simulink model "Orig_DSR_mod"  (R2021a)
settings: Solver=VariableStepAuto  StartTime=0.0  StopTime=10  RelTol=1e-3
values from neighbouring files (symbols this model uses):
  a = 0.5    [plot_3.m]
  alpha = 1.192    [plot_3.m]
  betac = 5    [plot_3.m]
  betacd = 3    [plot_3.m]
  c1 = 1    [plot_3.m]
  delay = 0.02    [plot_3.m]
  delay_a = 0.01    [plot_3.m]
  gnet = 0    [plot_3.m]
  omega = 5    [plot_3.m]
  omegader = 40    [plot_3.m]
libraries: cstblocks x37, simulink x4
(part 2 of 3)

== system Orig_DSR_mod/DSR_Input1/(I-beta*K)V_dot_est ==
  pos1 : Inport
  pos2 : Inport  Port=2
  pos3 : Inport  Port=3
  pos4 : Inport  Port=4
  pos5 : Inport  Port=5
  pos6 : Inport  Port=6
  pos1sense : Inport  Port=7
  pos2sense : Inport  Port=8
  pos3sense : Inport  Port=9
  pos4sense : Inport  Port=10
  pos5sense : Inport  Port=11
  pos6sense : Inport  Port=12
  (I-beta*K) : Subsystem
      settings: PortSchema="{\"entries\":[{\"content\":{\"sides\":[{\"content\":{\"connectorIds\":[\"In1\",\"In2\",\"In3\",\"In4\",\"In5\",\"In6\"]},\"type\":\"ConnectorPlacement.EquallySpacedRectSide\",\"uuid\":\"24ff0189-2e26-4de2-9c90-2043606e3d63\"},{\"content\":{\"connectorIds\":[\"Out1\",\"Out2\",\"Out3\",\"Out4\",\"Out5\",\"Out6\"],\"side\":\"RIGHT\"},\"type\":\"ConnectorPlacement.EquallySpacedRectSide\",\"uuid\":\"7efe01dd-8101-429e-adc6-a10b45356e48\"},{\"content\":{\"connectorIds\":[],\"side\":\"TOP\"},\"type\":\"ConnectorPlacement.EquallySpacedRectSide\",\"uuid\":\"5c1fc1f4-b8b0-4afd-80fe-11f4d157d0fc\"},{\"content\":{\"connectorIds\":[\"In7\",\"In8\",\"In9\",\"In10\",\"In11\",\"In12\"],\"side\":\"BOTTOM\"},\"type\":\"ConnectorPlacement.EquallySpacedRectSide\",\"uuid\":\"be77b686-a0b8-400e-8c92-c0517b137255\"}]},\"type\":\"ConnectorPlacement.EquallySpacedConnector\",\"uuid\":\"3e3502e3-b8a3-4e9d-9b78-ab08dd870d4b\"}],\"packageUris\":[\"http://schema.mathworks.com/mf0/Connector/R2020b\"],\"version\":\"1.0\"}"
  DerivativeEstimate : Subsystem
  DerivativeEstimate1 : Subsystem
  Output : Outport
  Output1 : Outport  Port=2
  Output2 : Outport  Port=3
  Output3 : Outport  Port=4
  Output4 : Outport  Port=5
  Output5 : Outport  Port=6
  wires:
  DerivativeEstimate/3(est2) -> (I-beta*K)/3(Input2)
  DerivativeEstimate/6(est5) -> (I-beta*K)/6(Input5)
  pos2/1 -> DerivativeEstimate/2(pos1)
  DerivativeEstimate/4(est3) -> (I-beta*K)/4(Input3)
  DerivativeEstimate/2(est1) -> (I-beta*K)/2(Input1)
  DerivativeEstimate/1(est) -> (I-beta*K)/1(Input)
  DerivativeEstimate/5(est4) -> (I-beta*K)/5(Input4)
  (I-beta*K)/6(Output5) -> Output5/1
  (I-beta*K)/3(Output2) -> Output2/1
  (I-beta*K)/4(Output3) -> Output3/1
  (I-beta*K)/5(Output4) -> Output4/1
  pos5/1 -> DerivativeEstimate/5(pos4)
  pos6/1 -> DerivativeEstimate/6(pos5)
  pos3/1 -> DerivativeEstimate/3(pos2)
  (I-beta*K)/2(Output1) -> Output1/1
  pos1/1 -> DerivativeEstimate/1(pos)
  pos4/1 -> DerivativeEstimate/4(pos3)
  (I-beta*K)/1(Output) -> Output/1
  pos1sense/1 -> DerivativeEstimate1/1(pos)
  pos2sense/1 -> DerivativeEstimate1/2(pos1)
  pos3sense/1 -> DerivativeEstimate1/3(pos2)
  pos4sense/1 -> DerivativeEstimate1/4(pos3)
  pos5sense/1 -> DerivativeEstimate1/5(pos4)
  pos6sense/1 -> DerivativeEstimate1/6(pos5)
  DerivativeEstimate1/1(est) -> (I-beta*K)/7(sense1)
  DerivativeEstimate1/2(est1) -> (I-beta*K)/8(sense2)
  DerivativeEstimate1/3(est2) -> (I-beta*K)/9(sense3)
  DerivativeEstimate1/4(est3) -> (I-beta*K)/10(sense4)
  DerivativeEstimate1/5(est4) -> (I-beta*K)/11(sense5)
  DerivativeEstimate1/6(est5) -> (I-beta*K)/12(sense6)

== system Orig_DSR_mod/DSR_Input1/Input Processor1 ==
  Input : Inport
  Derivative : Derivative
  Gain : Gain  Gain=alpha
  Gain1 : Gain  Gain=2
  Sum : Sum  Inputs=|++
  inputGain : Gain  Gain=alpha*betac
  Out1 : Outport
  wires:
  Gain1/1 -> Sum/2
  Derivative/1 -> Gain1/1
  Input/1 -> Gain/1, Derivative/1
  Sum/1 -> inputGain/1
  Gain/1 -> Sum/1
  inputGain/1 -> Out1/1

== system Orig_DSR_mod/DSR_Input1/KDgain1 ==
  Output : Inport
  Output1 : Inport  Port=2
  Output2 : Inport  Port=3
  Output3 : Inport  Port=4
  Output4 : Inport  Port=5
  Output5 : Inport  Port=6
  KDgain{1..3,8..10} (6 alike) : Gain  Gain=2*alpha*betac*c1
  u : Outport
  u1 : Outport  Port=2
  u2 : Outport  Port=3
  u3 : Outport  Port=4
  u4 : Outport  Port=5
  u5 : Outport  Port=6
  wires:
  Output2/1 -> KDgain8/1
  KDgain8/1 -> u2/1
  KDgain1/1 -> u1/1
  KDgain10/1 -> u4/1
  Output4/1 -> KDgain10/1
  Output/1 -> KDgain2/1
  KDgain2/1 -> u/1
  KDgain9/1 -> u3/1
  Output3/1 -> KDgain9/1
  KDgain3/1 -> u5/1
  Output5/1 -> KDgain3/1
  Output1/1 -> KDgain1/1

== system Orig_DSR_mod/DSR_Input1/KPgain1 ==
  Output : Inport
  Output1 : Inport  Port=2
  Output2 : Inport  Port=3
  Output3 : Inport  Port=4
  Output4 : Inport  Port=5
  Output5 : Inport  Port=6
  KPgain{1..6} (6 alike) : Gain  Gain=betac*c1*alpha^2
  Out1 : Outport
  Out2 : Outport  Port=2
  Out3 : Outport  Port=3
  Out4 : Outport  Port=4
  Out5 : Outport  Port=5
  Out6 : Outport  Port=6
  wires:
  Output4/1 -> KPgain5/1
  KPgain1/1 -> Out1/1
  KPgain2/1 -> Out2/1
  KPgain5/1 -> Out5/1
  Output/1 -> KPgain1/1
  Output3/1 -> KPgain4/1
  Output5/1 -> KPgain6/1
  Output1/1 -> KPgain2/1
  KPgain3/1 -> Out3/1
  KPgain6/1 -> Out6/1
  Output2/1 -> KPgain3/1
  KPgain4/1 -> Out4/1

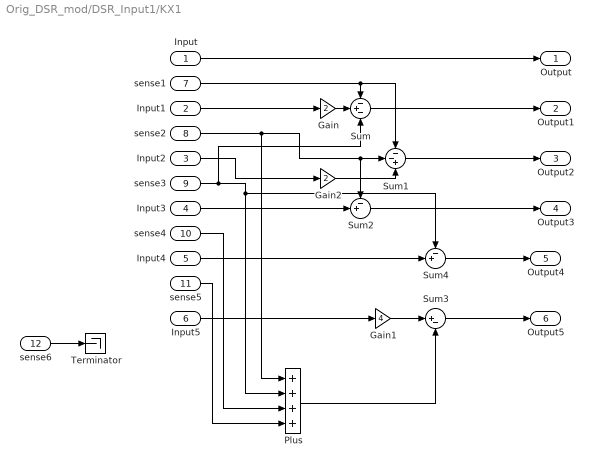
== system Orig_DSR_mod/DSR_Input1/KX1 ==
  Input : Inport
  Input1 : Inport  Port=2
  Input2 : Inport  Port=3
  Input3 : Inport  Port=4
  Input4 : Inport  Port=5
  Input5 : Inport  Port=6
  sense1 : Inport  Port=7
  sense2 : Inport  Port=8
  sense3 : Inport  Port=9
  sense4 : Inport  Port=10
  sense5 : Inport  Port=11
  sense6 : Inport  Port=12
  Gain : Gain  Gain=2
  Gain1 : Gain  Gain=4
  Gain2 : Gain  Gain=2
  Plus : Sum  Inputs=++++
  Sum : Sum  Inputs=-+-
  Sum1 : Sum  Inputs=--+
  Sum2 : Sum  Inputs=-+|
  Sum3 : Sum  Inputs=|+-
  Sum4 : Sum  Inputs=-+|
  Terminator : Terminator
  Output : Outport
  Output1 : Outport  Port=2
  Output2 : Outport  Port=3
  Output3 : Outport  Port=4
  Output4 : Outport  Port=5
  Output5 : Outport  Port=6
  wires:
  Input1/1 -> Gain/1
  Input/1 -> Output/1
  Input2/1 -> Gain2/1
  Sum1/1 -> Output2/1
  Input4/1 -> Sum4/2
  Gain/1 -> Sum/2
  Gain2/1 -> Sum1/3
  Sum/1 -> Output1/1
  Plus/1 -> Sum3/2
  Sum3/1 -> Output5/1
  Input5/1 -> Gain1/1
  Sum4/1 -> Output4/1
  Input3/1 -> Sum2/2
  Sum2/1 -> Output3/1
  Gain1/1 -> Sum3/1
  sense1/1 -> Sum1/1, Sum/1
  sense2/1 -> Sum2/1, Sum1/2, Plus/1
  sense3/1 -> Sum4/1, Plus/2, Sum/3
  sense4/1 -> Plus/3
  sense5/1 -> Plus/4
  sense6/1 -> Terminator/1

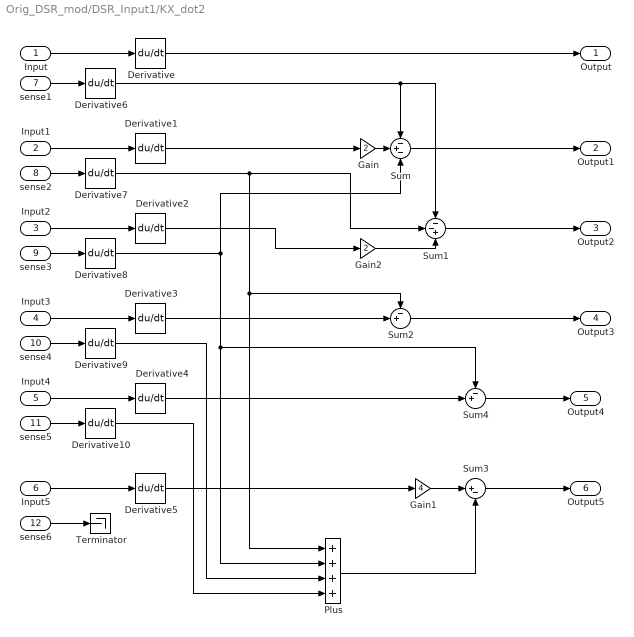
== system Orig_DSR_mod/DSR_Input1/KX_dot2 ==
  Input : Inport
  Input1 : Inport  Port=2
  Input2 : Inport  Port=3
  Input3 : Inport  Port=4
  Input4 : Inport  Port=5
  Input5 : Inport  Port=6
  sense1 : Inport  Port=7
  sense2 : Inport  Port=8
  sense3 : Inport  Port=9
  sense4 : Inport  Port=10
  sense5 : Inport  Port=11
  sense6 : Inport  Port=12
  Derivative{,1..10} (11 alike) : Derivative
  Gain : Gain  Gain=2
  Gain1 : Gain  Gain=4
  Gain2 : Gain  Gain=2
  Plus : Sum  Inputs=++++
  Sum : Sum  Inputs=-+-
  Sum1 : Sum  Inputs=--+
  Sum2 : Sum  Inputs=-+|
  Sum3 : Sum  Inputs=|+-
  Sum4 : Sum  Inputs=-+|
  Terminator : Terminator
  Output : Outport
  Output1 : Outport  Port=2
  Output2 : Outport  Port=3
  Output3 : Outport  Port=4
  Output4 : Outport  Port=5
  Output5 : Outport  Port=6
  wires:
  Input1/1 -> Derivative1/1
  Input/1 -> Derivative/1
  Input2/1 -> Derivative2/1
  Sum1/1 -> Output2/1
  Input4/1 -> Derivative4/1
  Gain/1 -> Sum/2
  Gain2/1 -> Sum1/3
  Sum/1 -> Output1/1
  Plus/1 -> Sum3/2
  Sum3/1 -> Output5/1
  Input5/1 -> Derivative5/1
  Sum4/1 -> Output4/1
  Input3/1 -> Derivative3/1
  Sum2/1 -> Output3/1
  Gain1/1 -> Sum3/1
  Derivative1/1 -> Gain/1
  Derivative2/1 -> Gain2/1
  Derivative3/1 -> Sum2/2
  Derivative4/1 -> Sum4/2
  Derivative5/1 -> Gain1/1
  sense1/1 -> Derivative6/1
  sense2/1 -> Derivative7/1
  sense3/1 -> Derivative8/1
  sense4/1 -> Derivative9/1
  sense5/1 -> Derivative10/1
  Derivative/1 -> Output/1
  Derivative6/1 -> Sum/1, Sum1/1
  Derivative7/1 -> Sum1/2, Sum2/1, Plus/1
  Derivative8/1 -> Sum4/1, Plus/2, Sum/3
  Derivative9/1 -> Plus/3
  Derivative10/1 -> Plus/4
  sense6/1 -> Terminator/1

== system Orig_DSR_mod/DSR_Input1/Subsystem1 ==
  u : Inport
  u1 : Inport  Port=2
  u2 : Inport  Port=3
  u3 : Inport  Port=4
  u4 : Inport  Port=5
  u5 : Inport  Port=6
  Varying Lowpass Filter{,1..5} (6 alike) : cstblocks/Linear Parameter Varying/Varying Lowpass Filter  N=1
  Zero : Constant  Value=omegader  OutDataTypeStr=Inherit: Inherit via back propagation
  Out7 : Outport
  Out8 : Outport  Port=2
  Out9 : Outport  Port=3
  Out10 : Outport  Port=4
  Out11 : Outport  Port=5
  Out12 : Outport  Port=6
  wires:
  u/1 -> Varying Lowpass Filter/1
  u1/1 -> Varying Lowpass Filter1/1
  u2/1 -> Varying Lowpass Filter2/1
  u5/1 -> Varying Lowpass Filter5/1
  u3/1 -> Varying Lowpass Filter3/1
  Zero/1 -> Varying Lowpass Filter5/2, Varying Lowpass Filter4/2, Varying Lowpass Filter2/2, Varying Lowpass Filter1/2, Varying Lowpass Filter/2, Varying Lowpass Filter3/2
  Varying Lowpass Filter5/1 -> Out12/1
  u4/1 -> Varying Lowpass Filter4/1
  Varying Lowpass Filter/1 -> Out7/1
  Varying Lowpass Filter4/1 -> Out11/1
  Varying Lowpass Filter1/1 -> Out8/1
  Varying Lowpass Filter2/1 -> Out9/1
  Varying Lowpass Filter3/1 -> Out10/1

== system Orig_DSR_mod/DSR_Input2/(I-beta*K)V_dot_est ==
  pos1 : Inport
  pos2 : Inport  Port=2
  pos3 : Inport  Port=3
  pos4 : Inport  Port=4
  pos5 : Inport  Port=5
  pos6 : Inport  Port=6
  pos1sense : Inport  Port=7
  pos2sense : Inport  Port=8
  pos3sense : Inport  Port=9
  pos4sense : Inport  Port=10
  pos5sense : Inport  Port=11
  pos6sense : Inport  Port=12
  (I-beta*K) : Subsystem
      settings: PortSchema="{\"entries\":[{\"content\":{\"sides\":[{\"content\":{\"connectorIds\":[\"In1\",\"In2\",\"In3\",\"In4\",\"In5\",\"In6\"]},\"type\":\"ConnectorPlacement.EquallySpacedRectSide\",\"uuid\":\"24ff0189-2e26-4de2-9c90-2043606e3d63\"},{\"content\":{\"connectorIds\":[\"Out1\",\"Out2\",\"Out3\",\"Out4\",\"Out5\",\"Out6\"],\"side\":\"RIGHT\"},\"type\":\"ConnectorPlacement.EquallySpacedRectSide\",\"uuid\":\"7efe01dd-8101-429e-adc6-a10b45356e48\"},{\"content\":{\"connectorIds\":[],\"side\":\"TOP\"},\"type\":\"ConnectorPlacement.EquallySpacedRectSide\",\"uuid\":\"5c1fc1f4-b8b0-4afd-80fe-11f4d157d0fc\"},{\"content\":{\"connectorIds\":[\"In7\",\"In8\",\"In9\",\"In10\",\"In11\",\"In12\"],\"side\":\"BOTTOM\"},\"type\":\"ConnectorPlacement.EquallySpacedRectSide\",\"uuid\":\"be77b686-a0b8-400e-8c92-c0517b137255\"}]},\"type\":\"ConnectorPlacement.EquallySpacedConnector\",\"uuid\":\"3e3502e3-b8a3-4e9d-9b78-ab08dd870d4b\"}],\"packageUris\":[\"http://schema.mathworks.com/mf0/Connector/R2020b\"],\"version\":\"1.0\"}"
  DerivativeEstimate : Subsystem
  DerivativeEstimate1 : Subsystem
  Output : Outport
  Output1 : Outport  Port=2
  Output2 : Outport  Port=3
  Output3 : Outport  Port=4
  Output4 : Outport  Port=5
  Output5 : Outport  Port=6
  wires:
  DerivativeEstimate/3(est2) -> (I-beta*K)/3(Input2)
  DerivativeEstimate/6(est5) -> (I-beta*K)/6(Input5)
  pos2/1 -> DerivativeEstimate/2(pos1)
  DerivativeEstimate/4(est3) -> (I-beta*K)/4(Input3)
  DerivativeEstimate/2(est1) -> (I-beta*K)/2(Input1)
  DerivativeEstimate/1(est) -> (I-beta*K)/1(Input)
  DerivativeEstimate/5(est4) -> (I-beta*K)/5(Input4)
  (I-beta*K)/6(Output5) -> Output5/1
  (I-beta*K)/3(Output2) -> Output2/1
  (I-beta*K)/4(Output3) -> Output3/1
  (I-beta*K)/5(Output4) -> Output4/1
  pos5/1 -> DerivativeEstimate/5(pos4)
  pos6/1 -> DerivativeEstimate/6(pos5)
  pos3/1 -> DerivativeEstimate/3(pos2)
  (I-beta*K)/2(Output1) -> Output1/1
  pos1/1 -> DerivativeEstimate/1(pos)
  pos4/1 -> DerivativeEstimate/4(pos3)
  (I-beta*K)/1(Output) -> Output/1
  pos1sense/1 -> DerivativeEstimate1/1(pos)
  pos2sense/1 -> DerivativeEstimate1/2(pos1)
  pos3sense/1 -> DerivativeEstimate1/3(pos2)
  pos4sense/1 -> DerivativeEstimate1/4(pos3)
  pos5sense/1 -> DerivativeEstimate1/5(pos4)
  pos6sense/1 -> DerivativeEstimate1/6(pos5)
  DerivativeEstimate1/1(est) -> (I-beta*K)/7(sense1)
  DerivativeEstimate1/2(est1) -> (I-beta*K)/8(sense2)
  DerivativeEstimate1/3(est2) -> (I-beta*K)/9(sense3)
  DerivativeEstimate1/4(est3) -> (I-beta*K)/10(sense4)
  DerivativeEstimate1/5(est4) -> (I-beta*K)/11(sense5)
  DerivativeEstimate1/6(est5) -> (I-beta*K)/12(sense6)

== system Orig_DSR_mod/DSR_Input2/Input Processor1 ==
  Input : Inport
  Derivative : Derivative
  Gain : Gain  Gain=alpha
  Gain1 : Gain  Gain=2
  Sum : Sum  Inputs=|++
  inputGain : Gain  Gain=alpha*betac*c1
  Out1 : Outport
  wires:
  Gain1/1 -> Sum/2
  Derivative/1 -> Gain1/1
  Input/1 -> Gain/1, Derivative/1
  Sum/1 -> inputGain/1
  Gain/1 -> Sum/1
  inputGain/1 -> Out1/1

== system Orig_DSR_mod/DSR_Input2/KDgain1 ==
  Output : Inport
  Output1 : Inport  Port=2
  Output2 : Inport  Port=3
  Output3 : Inport  Port=4
  Output4 : Inport  Port=5
  Output5 : Inport  Port=6
  KDgain{1..3,8..10} (6 alike) : Gain  Gain=2*alpha*betac*c1
  u : Outport
  u1 : Outport  Port=2
  u2 : Outport  Port=3
  u3 : Outport  Port=4
  u4 : Outport  Port=5
  u5 : Outport  Port=6
  wires:
  Output2/1 -> KDgain8/1
  KDgain8/1 -> u2/1
  KDgain1/1 -> u1/1
  KDgain10/1 -> u4/1
  Output4/1 -> KDgain10/1
  Output/1 -> KDgain2/1
  KDgain2/1 -> u/1
  KDgain9/1 -> u3/1
  Output3/1 -> KDgain9/1
  KDgain3/1 -> u5/1
  Output5/1 -> KDgain3/1
  Output1/1 -> KDgain1/1

== system Orig_DSR_mod/DSR_Input2/KPgain1 ==
  Output : Inport
  Output1 : Inport  Port=2
  Output2 : Inport  Port=3
  Output3 : Inport  Port=4
  Output4 : Inport  Port=5
  Output5 : Inport  Port=6
  KPgain{1..6} (6 alike) : Gain  Gain=betac*c1*alpha^2
  Out1 : Outport
  Out2 : Outport  Port=2
  Out3 : Outport  Port=3
  Out4 : Outport  Port=4
  Out5 : Outport  Port=5
  Out6 : Outport  Port=6
  wires:
  Output4/1 -> KPgain5/1
  KPgain1/1 -> Out1/1
  KPgain2/1 -> Out2/1
  KPgain5/1 -> Out5/1
  Output/1 -> KPgain1/1
  Output3/1 -> KPgain4/1
  Output5/1 -> KPgain6/1
  Output1/1 -> KPgain2/1
  KPgain3/1 -> Out3/1
  KPgain6/1 -> Out6/1
  Output2/1 -> KPgain3/1
  KPgain4/1 -> Out4/1

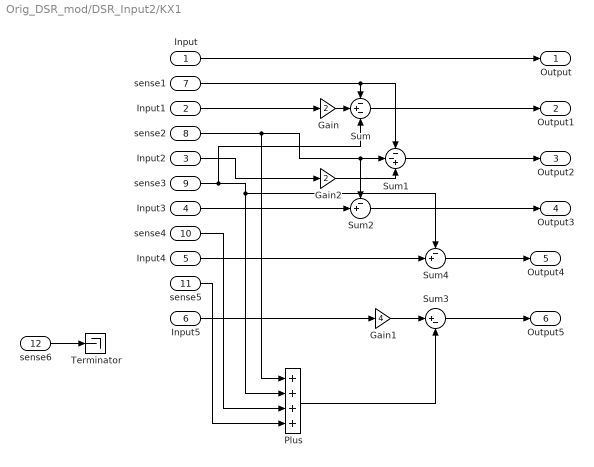
== system Orig_DSR_mod/DSR_Input2/KX1 ==
  Input : Inport
  Input1 : Inport  Port=2
  Input2 : Inport  Port=3
  Input3 : Inport  Port=4
  Input4 : Inport  Port=5
  Input5 : Inport  Port=6
  sense1 : Inport  Port=7
  sense2 : Inport  Port=8
  sense3 : Inport  Port=9
  sense4 : Inport  Port=10
  sense5 : Inport  Port=11
  sense6 : Inport  Port=12
  Gain : Gain  Gain=2
  Gain1 : Gain  Gain=4
  Gain2 : Gain  Gain=2
  Plus : Sum  Inputs=++++
  Sum : Sum  Inputs=-+-
  Sum1 : Sum  Inputs=--+
  Sum2 : Sum  Inputs=-+|
  Sum3 : Sum  Inputs=|+-
  Sum4 : Sum  Inputs=-+|
  Terminator : Terminator
  Output : Outport
  Output1 : Outport  Port=2
  Output2 : Outport  Port=3
  Output3 : Outport  Port=4
  Output4 : Outport  Port=5
  Output5 : Outport  Port=6
  wires:
  Input1/1 -> Gain/1
  Input/1 -> Output/1
  Input2/1 -> Gain2/1
  Sum1/1 -> Output2/1
  Input4/1 -> Sum4/2
  Gain/1 -> Sum/2
  Gain2/1 -> Sum1/3
  Sum/1 -> Output1/1
  Plus/1 -> Sum3/2
  Sum3/1 -> Output5/1
  Input5/1 -> Gain1/1
  Sum4/1 -> Output4/1
  Input3/1 -> Sum2/2
  Sum2/1 -> Output3/1
  Gain1/1 -> Sum3/1
  sense1/1 -> Sum1/1, Sum/1
  sense2/1 -> Sum2/1, Sum1/2, Plus/1
  sense3/1 -> Sum4/1, Plus/2, Sum/3
  sense4/1 -> Plus/3
  sense5/1 -> Plus/4
  sense6/1 -> Terminator/1

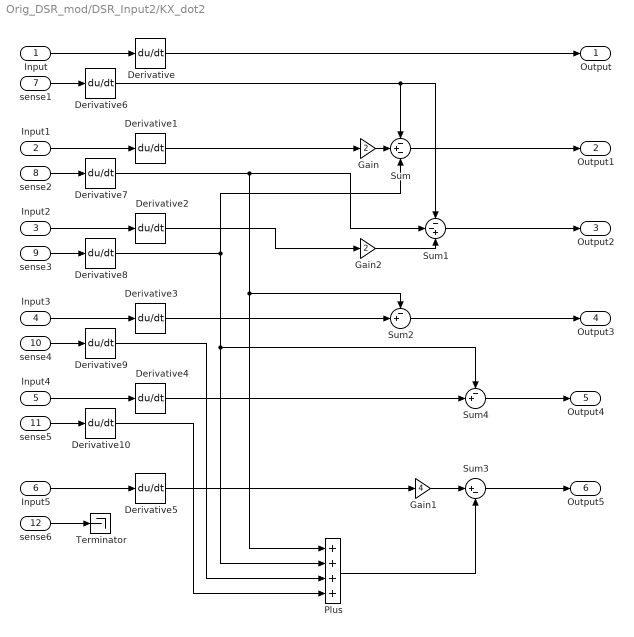
== system Orig_DSR_mod/DSR_Input2/KX_dot2 ==
  Input : Inport
  Input1 : Inport  Port=2
  Input2 : Inport  Port=3
  Input3 : Inport  Port=4
  Input4 : Inport  Port=5
  Input5 : Inport  Port=6
  sense1 : Inport  Port=7
  sense2 : Inport  Port=8
  sense3 : Inport  Port=9
  sense4 : Inport  Port=10
  sense5 : Inport  Port=11
  sense6 : Inport  Port=12
  Derivative{,1..10} (11 alike) : Derivative
  Gain : Gain  Gain=2
  Gain1 : Gain  Gain=4
  Gain2 : Gain  Gain=2
  Plus : Sum  Inputs=++++
  Sum : Sum  Inputs=-+-
  Sum1 : Sum  Inputs=--+
  Sum2 : Sum  Inputs=-+|
  Sum3 : Sum  Inputs=|+-
  Sum4 : Sum  Inputs=-+|
  Terminator : Terminator
  Output : Outport
  Output1 : Outport  Port=2
  Output2 : Outport  Port=3
  Output3 : Outport  Port=4
  Output4 : Outport  Port=5
  Output5 : Outport  Port=6
  wires:
  Input1/1 -> Derivative1/1
  Input/1 -> Derivative/1
  Input2/1 -> Derivative2/1
  Sum1/1 -> Output2/1
  Input4/1 -> Derivative4/1
  Gain/1 -> Sum/2
  Gain2/1 -> Sum1/3
  Sum/1 -> Output1/1
  Plus/1 -> Sum3/2
  Sum3/1 -> Output5/1
  Input5/1 -> Derivative5/1
  Sum4/1 -> Output4/1
  Input3/1 -> Derivative3/1
  Sum2/1 -> Output3/1
  Gain1/1 -> Sum3/1
  Derivative1/1 -> Gain/1
  Derivative2/1 -> Gain2/1
  Derivative3/1 -> Sum2/2
  Derivative4/1 -> Sum4/2
  Derivative5/1 -> Gain1/1
  sense1/1 -> Derivative6/1
  sense2/1 -> Derivative7/1
  sense3/1 -> Derivative8/1
  sense4/1 -> Derivative9/1
  sense5/1 -> Derivative10/1
  Derivative/1 -> Output/1
  Derivative6/1 -> Sum/1, Sum1/1
  Derivative7/1 -> Sum1/2, Sum2/1, Plus/1
  Derivative8/1 -> Sum4/1, Plus/2, Sum/3
  Derivative9/1 -> Plus/3
  Derivative10/1 -> Plus/4
  sense6/1 -> Terminator/1

== system Orig_DSR_mod/DSR_Input2/Subsystem1 ==
  u : Inport
  u1 : Inport  Port=2
  u2 : Inport  Port=3
  u3 : Inport  Port=4
  u4 : Inport  Port=5
  u5 : Inport  Port=6
  Varying Lowpass Filter{,1..5} (6 alike) : cstblocks/Linear Parameter Varying/Varying Lowpass Filter  N=1
  Zero : Constant  Value=omegader  OutDataTypeStr=Inherit: Inherit via back propagation
  Out7 : Outport
  Out8 : Outport  Port=2
  Out9 : Outport  Port=3
  Out10 : Outport  Port=4
  Out11 : Outport  Port=5
  Out12 : Outport  Port=6
  wires:
  u/1 -> Varying Lowpass Filter/1
  u1/1 -> Varying Lowpass Filter1/1
  u2/1 -> Varying Lowpass Filter2/1
  u5/1 -> Varying Lowpass Filter5/1
  u3/1 -> Varying Lowpass Filter3/1
  Zero/1 -> Varying Lowpass Filter5/2, Varying Lowpass Filter4/2, Varying Lowpass Filter2/2, Varying Lowpass Filter1/2, Varying Lowpass Filter/2, Varying Lowpass Filter3/2
  Varying Lowpass Filter5/1 -> Out12/1
  u4/1 -> Varying Lowpass Filter4/1
  Varying Lowpass Filter/1 -> Out7/1
  Varying Lowpass Filter4/1 -> Out11/1
  Varying Lowpass Filter1/1 -> Out8/1
  Varying Lowpass Filter2/1 -> Out9/1
  Varying Lowpass Filter3/1 -> Out10/1

== system Orig_DSR_mod/DSR_Input3/(I-beta*K)V_dot_est ==
  pos1 : Inport
  pos2 : Inport  Port=2
  pos3 : Inport  Port=3
  pos4 : Inport  Port=4
  pos5 : Inport  Port=5
  pos6 : Inport  Port=6
  pos1sense : Inport  Port=7
  pos2sense : Inport  Port=8
  pos3sense : Inport  Port=9
  pos4sense : Inport  Port=10
  pos5sense : Inport  Port=11
  pos6sense : Inport  Port=12
  (I-beta*K) : Subsystem
      settings: PortSchema="{\"entries\":[{\"content\":{\"sides\":[{\"content\":{\"connectorIds\":[\"In1\",\"In2\",\"In3\",\"In4\",\"In5\",\"In6\"]},\"type\":\"ConnectorPlacement.EquallySpacedRectSide\",\"uuid\":\"24ff0189-2e26-4de2-9c90-2043606e3d63\"},{\"content\":{\"connectorIds\":[\"Out1\",\"Out2\",\"Out3\",\"Out4\",\"Out5\",\"Out6\"],\"side\":\"RIGHT\"},\"type\":\"ConnectorPlacement.EquallySpacedRectSide\",\"uuid\":\"7efe01dd-8101-429e-adc6-a10b45356e48\"},{\"content\":{\"connectorIds\":[],\"side\":\"TOP\"},\"type\":\"ConnectorPlacement.EquallySpacedRectSide\",\"uuid\":\"5c1fc1f4-b8b0-4afd-80fe-11f4d157d0fc\"},{\"content\":{\"connectorIds\":[\"In7\",\"In8\",\"In9\",\"In10\",\"In11\",\"In12\"],\"side\":\"BOTTOM\"},\"type\":\"ConnectorPlacement.EquallySpacedRectSide\",\"uuid\":\"be77b686-a0b8-400e-8c92-c0517b137255\"}]},\"type\":\"ConnectorPlacement.EquallySpacedConnector\",\"uuid\":\"3e3502e3-b8a3-4e9d-9b78-ab08dd870d4b\"}],\"packageUris\":[\"http://schema.mathworks.com/mf0/Connector/R2020b\"],\"version\":\"1.0\"}"
  DerivativeEstimate : Subsystem
  DerivativeEstimate1 : Subsystem
  Output : Outport
  Output1 : Outport  Port=2
  Output2 : Outport  Port=3
  Output3 : Outport  Port=4
  Output4 : Outport  Port=5
  Output5 : Outport  Port=6
  wires:
  DerivativeEstimate/3(est2) -> (I-beta*K)/3(Input2)
  DerivativeEstimate/6(est5) -> (I-beta*K)/6(Input5)
  pos2/1 -> DerivativeEstimate/2(pos1)
  DerivativeEstimate/4(est3) -> (I-beta*K)/4(Input3)
  DerivativeEstimate/2(est1) -> (I-beta*K)/2(Input1)
  DerivativeEstimate/1(est) -> (I-beta*K)/1(Input)
  DerivativeEstimate/5(est4) -> (I-beta*K)/5(Input4)
  (I-beta*K)/6(Output5) -> Output5/1
  (I-beta*K)/3(Output2) -> Output2/1
  (I-beta*K)/4(Output3) -> Output3/1
  (I-beta*K)/5(Output4) -> Output4/1
  pos5/1 -> DerivativeEstimate/5(pos4)
  pos6/1 -> DerivativeEstimate/6(pos5)
  pos3/1 -> DerivativeEstimate/3(pos2)
  (I-beta*K)/2(Output1) -> Output1/1
  pos1/1 -> DerivativeEstimate/1(pos)
  pos4/1 -> DerivativeEstimate/4(pos3)
  (I-beta*K)/1(Output) -> Output/1
  pos1sense/1 -> DerivativeEstimate1/1(pos)
  pos2sense/1 -> DerivativeEstimate1/2(pos1)
  pos3sense/1 -> DerivativeEstimate1/3(pos2)
  pos4sense/1 -> DerivativeEstimate1/4(pos3)
  pos5sense/1 -> DerivativeEstimate1/5(pos4)
  pos6sense/1 -> DerivativeEstimate1/6(pos5)
  DerivativeEstimate1/1(est) -> (I-beta*K)/7(sense1)
  DerivativeEstimate1/2(est1) -> (I-beta*K)/8(sense2)
  DerivativeEstimate1/3(est2) -> (I-beta*K)/9(sense3)
  DerivativeEstimate1/4(est3) -> (I-beta*K)/10(sense4)
  DerivativeEstimate1/5(est4) -> (I-beta*K)/11(sense5)
  DerivativeEstimate1/6(est5) -> (I-beta*K)/12(sense6)

== system Orig_DSR_mod/DSR_Input3/Input Processor1 ==
  Input : Inport
  Derivative : Derivative
  Gain : Gain  Gain=alpha
  Gain1 : Gain  Gain=2
  Sum : Sum  Inputs=|++
  Varying Lowpass Filter : cstblocks/Linear Parameter Varying/Varying Lowpass Filter  N=1
  Zero : Constant  Value=omegader  OutDataTypeStr=Inherit: Inherit via back propagation
  inputGain : Gain  Gain=alpha*betac
  Out1 : Outport
  wires:
  Gain1/1 -> Sum/2
  Varying Lowpass Filter/1 -> Gain1/1
  Input/1 -> Derivative/1, Gain/1
  Sum/1 -> inputGain/1
  Gain/1 -> Sum/1
  inputGain/1 -> Out1/1
  Zero/1 -> Varying Lowpass Filter/2
  Derivative/1 -> Varying Lowpass Filter/1

== system Orig_DSR_mod/DSR_Input3/KDgain1 ==
  Output : Inport
  Output1 : Inport  Port=2
  Output2 : Inport  Port=3
  Output3 : Inport  Port=4
  Output4 : Inport  Port=5
  Output5 : Inport  Port=6
  KDgain{1..3,8..10} (6 alike) : Gain  Gain=2*alpha*betac*c1
  u : Outport
  u1 : Outport  Port=2
  u2 : Outport  Port=3
  u3 : Outport  Port=4
  u4 : Outport  Port=5
  u5 : Outport  Port=6
  wires:
  Output2/1 -> KDgain8/1
  KDgain8/1 -> u2/1
  KDgain1/1 -> u1/1
  KDgain10/1 -> u4/1
  Output4/1 -> KDgain10/1
  Output/1 -> KDgain2/1
  KDgain2/1 -> u/1
  KDgain9/1 -> u3/1
  Output3/1 -> KDgain9/1
  KDgain3/1 -> u5/1
  Output5/1 -> KDgain3/1
  Output1/1 -> KDgain1/1

== system Orig_DSR_mod/DSR_Input3/KPgain1 ==
  Output : Inport
  Output1 : Inport  Port=2
  Output2 : Inport  Port=3
  Output3 : Inport  Port=4
  Output4 : Inport  Port=5
  Output5 : Inport  Port=6
  KPgain{1..6} (6 alike) : Gain  Gain=betac*c1*alpha^2
  Out1 : Outport
  Out2 : Outport  Port=2
  Out3 : Outport  Port=3
  Out4 : Outport  Port=4
  Out5 : Outport  Port=5
  Out6 : Outport  Port=6
  wires:
  Output4/1 -> KPgain5/1
  KPgain1/1 -> Out1/1
  KPgain2/1 -> Out2/1
  KPgain5/1 -> Out5/1
  Output/1 -> KPgain1/1
  Output3/1 -> KPgain4/1
  Output5/1 -> KPgain6/1
  Output1/1 -> KPgain2/1
  KPgain3/1 -> Out3/1
  KPgain6/1 -> Out6/1
  Output2/1 -> KPgain3/1
  KPgain4/1 -> Out4/1

== system Orig_DSR_mod/DSR_Input3/KX1 ==
  Input : Inport
  Input1 : Inport  Port=2
  Input2 : Inport  Port=3
  Input3 : Inport  Port=4
  Input4 : Inport  Port=5
  Input5 : Inport  Port=6
  sense1 : Inport  Port=7
  sense2 : Inport  Port=8
  sense3 : Inport  Port=9
  sense4 : Inport  Port=10
  sense5 : Inport  Port=11
  sense6 : Inport  Port=12
  Gain : Gain  Gain=2
  Gain1 : Gain  Gain=4
  Gain2 : Gain  Gain=2
  Plus : Sum  Inputs=++++
  Sum : Sum  Inputs=-+-
  Sum1 : Sum  Inputs=--+
  Sum2 : Sum  Inputs=-+|
  Sum3 : Sum  Inputs=|+-
  Sum4 : Sum  Inputs=-+|
  Terminator : Terminator
  Output : Outport
  Output1 : Outport  Port=2
  Output2 : Outport  Port=3
  Output3 : Outport  Port=4
  Output4 : Outport  Port=5
  Output5 : Outport  Port=6
  wires:
  Input1/1 -> Gain/1
  Input/1 -> Output/1
  Input2/1 -> Gain2/1
  Sum1/1 -> Output2/1
  Input4/1 -> Sum4/2
  Gain/1 -> Sum/2
  Gain2/1 -> Sum1/3
  Sum/1 -> Output1/1
  Plus/1 -> Sum3/2
  Sum3/1 -> Output5/1
  Input5/1 -> Gain1/1
  Sum4/1 -> Output4/1
  Input3/1 -> Sum2/2
  Sum2/1 -> Output3/1
  Gain1/1 -> Sum3/1
  sense1/1 -> Sum1/1, Sum/1
  sense2/1 -> Sum2/1, Sum1/2, Plus/1
  sense3/1 -> Sum4/1, Plus/2, Sum/3
  sense4/1 -> Plus/3
  sense5/1 -> Plus/4
  sense6/1 -> Terminator/1

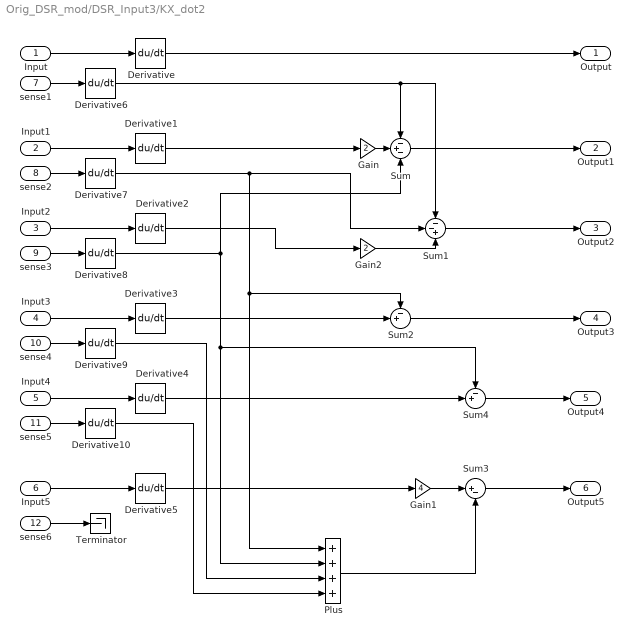
== system Orig_DSR_mod/DSR_Input3/KX_dot2 ==
  Input : Inport
  Input1 : Inport  Port=2
  Input2 : Inport  Port=3
  Input3 : Inport  Port=4
  Input4 : Inport  Port=5
  Input5 : Inport  Port=6
  sense1 : Inport  Port=7
  sense2 : Inport  Port=8
  sense3 : Inport  Port=9
  sense4 : Inport  Port=10
  sense5 : Inport  Port=11
  sense6 : Inport  Port=12
  Derivative{,1..10} (11 alike) : Derivative
  Gain : Gain  Gain=2
  Gain1 : Gain  Gain=4
  Gain2 : Gain  Gain=2
  Plus : Sum  Inputs=++++
  Sum : Sum  Inputs=-+-
  Sum1 : Sum  Inputs=--+
  Sum2 : Sum  Inputs=-+|
  Sum3 : Sum  Inputs=|+-
  Sum4 : Sum  Inputs=-+|
  Terminator : Terminator
  Output : Outport
  Output1 : Outport  Port=2
  Output2 : Outport  Port=3
  Output3 : Outport  Port=4
  Output4 : Outport  Port=5
  Output5 : Outport  Port=6
  wires:
  Input1/1 -> Derivative1/1
  Input/1 -> Derivative/1
  Input2/1 -> Derivative2/1
  Sum1/1 -> Output2/1
  Input4/1 -> Derivative4/1
  Gain/1 -> Sum/2
  Gain2/1 -> Sum1/3
  Sum/1 -> Output1/1
  Plus/1 -> Sum3/2
  Sum3/1 -> Output5/1
  Input5/1 -> Derivative5/1
  Sum4/1 -> Output4/1
  Input3/1 -> Derivative3/1
  Sum2/1 -> Output3/1
  Gain1/1 -> Sum3/1
  Derivative1/1 -> Gain/1
  Derivative2/1 -> Gain2/1
  Derivative3/1 -> Sum2/2
  Derivative4/1 -> Sum4/2
  Derivative5/1 -> Gain1/1
  sense1/1 -> Derivative6/1
  sense2/1 -> Derivative7/1
  sense3/1 -> Derivative8/1
  sense4/1 -> Derivative9/1
  sense5/1 -> Derivative10/1
  Derivative/1 -> Output/1
  Derivative6/1 -> Sum/1, Sum1/1
  Derivative7/1 -> Sum1/2, Sum2/1, Plus/1
  Derivative8/1 -> Sum4/1, Plus/2, Sum/3
  Derivative9/1 -> Plus/3
  Derivative10/1 -> Plus/4
  sense6/1 -> Terminator/1

== system Orig_DSR_mod/DSR_Input3/Subsystem1 ==
  u : Inport
  u1 : Inport  Port=2
  u2 : Inport  Port=3
  u3 : Inport  Port=4
  u4 : Inport  Port=5
  u5 : Inport  Port=6
  Varying Lowpass Filter{,1..5} (6 alike) : cstblocks/Linear Parameter Varying/Varying Lowpass Filter  N=1
  Zero : Constant  Value=omegader  OutDataTypeStr=Inherit: Inherit via back propagation
  Out7 : Outport
  Out8 : Outport  Port=2
  Out9 : Outport  Port=3
  Out10 : Outport  Port=4
  Out11 : Outport  Port=5
  Out12 : Outport  Port=6
  wires:
  u/1 -> Varying Lowpass Filter/1
  u1/1 -> Varying Lowpass Filter1/1
  u2/1 -> Varying Lowpass Filter2/1
  u5/1 -> Varying Lowpass Filter5/1
  u3/1 -> Varying Lowpass Filter3/1
  Zero/1 -> Varying Lowpass Filter5/2, Varying Lowpass Filter4/2, Varying Lowpass Filter2/2, Varying Lowpass Filter1/2, Varying Lowpass Filter/2, Varying Lowpass Filter3/2
  Varying Lowpass Filter5/1 -> Out12/1
  u4/1 -> Varying Lowpass Filter4/1
  Varying Lowpass Filter4/1 -> Out11/1
  Varying Lowpass Filter1/1 -> Out8/1
  Varying Lowpass Filter2/1 -> Out9/1
  Varying Lowpass Filter3/1 -> Out10/1
  Varying Lowpass Filter/1 -> Out7/1

== system Orig_DSR_mod/Max Deflection1/Average ==
  In1 : Inport
  In2 : Inport  Port=2
  In3 : Inport  Port=3
  In4 : Inport  Port=4
  In5 : Inport  Port=5
  In6 : Inport  Port=6
  Gain : Gain  Gain=1/6
  Sum10 : Sum  Inputs=++++++
  Out1 : Outport
  wires:
  In1/1 -> Sum10/1
  Sum10/1 -> Gain/1
  In3/1 -> Sum10/3
  In6/1 -> Sum10/6
  In4/1 -> Sum10/4
  Gain/1 -> Out1/1
  In5/1 -> Sum10/5
  In2/1 -> Sum10/2

== system Orig_DSR_mod/Max Deflection2/Average ==
  In1 : Inport
  In2 : Inport  Port=2
  In3 : Inport  Port=3
  In4 : Inport  Port=4
  In5 : Inport  Port=5
  In6 : Inport  Port=6
  Gain : Gain  Gain=1/6
  Sum10 : Sum  Inputs=++++++
  Out1 : Outport
  wires:
  In1/1 -> Sum10/1
  Sum10/1 -> Gain/1
  In3/1 -> Sum10/3
  In6/1 -> Sum10/6
  In4/1 -> Sum10/4
  Gain/1 -> Out1/1
  In5/1 -> Sum10/5
  In2/1 -> Sum10/2

== system Orig_DSR_mod/Max Deflection3/Average ==
  In1 : Inport
  In2 : Inport  Port=2
  In3 : Inport  Port=3
  In4 : Inport  Port=4
  In5 : Inport  Port=5
  In6 : Inport  Port=6
  Gain : Gain  Gain=1/6
  Sum10 : Sum  Inputs=++++++
  Out1 : Outport
  wires:
  In1/1 -> Sum10/1
  Sum10/1 -> Gain/1
  In3/1 -> Sum10/3
  In6/1 -> Sum10/6
  In4/1 -> Sum10/4
  Gain/1 -> Out1/1
  In5/1 -> Sum10/5
  In2/1 -> Sum10/2

== system Orig_DSR_mod/CDOB_Subsys1/ND/CDOB1 ==
  XRes : Inport
  Acc. : Inport  Port=2
  Derivative : Derivative  CoefficientInTFapproximation=0
  Gain : Gain  Gain=gnet/a
  Sum : Sum  Inputs=-+|
  Sum8 : Sum  Inputs=+-+
  Transfer Fcn2 : TransferFcn  Numerator=[gnet]  Denominator=[1 gnet]
  Dobsv : Outport
  wires:
  Transfer Fcn2/1 -> Sum/2
  Sum8/1 -> Transfer Fcn2/1
  Derivative/1 -> Sum8/2, Gain/1
  Gain/1 -> Sum8/1, Sum/1
  Sum/1 -> Dobsv/1
  XRes/1 -> Derivative/1
  Acc./1 -> Sum8/3

== system Orig_DSR_mod/CDOB_Subsys1/ND/TimeDelayComp ==
  SysOut : Inport
  Dobsv : Inport  Port=2
  DelayCom : TransferFcn  Numerator=[a]  Denominator=[1 a 0]
  Sum8 : Sum  Inputs=|++
  FeedBack : Outport
  wires:
  DelayCom/1 -> Sum8/2
  SysOut/1 -> Sum8/1
  Sum8/1 -> FeedBack/1
  Dobsv/1 -> DelayCom/1

== system Orig_DSR_mod/CDOB_Subsys1/ND1/CDOB1 ==
  XRes : Inport
  Acc. : Inport  Port=2
  Derivative : Derivative  CoefficientInTFapproximation=0
  Gain : Gain  Gain=gnet/a
  Sum : Sum  Inputs=-+|
  Sum8 : Sum  Inputs=+-+
  Transfer Fcn2 : TransferFcn  Numerator=[gnet]  Denominator=[1 gnet]
  Dobsv : Outport
  wires:
  Transfer Fcn2/1 -> Sum/2
  Sum8/1 -> Transfer Fcn2/1
  Derivative/1 -> Sum8/2, Gain/1
  Gain/1 -> Sum8/1, Sum/1
  Sum/1 -> Dobsv/1
  XRes/1 -> Derivative/1
  Acc./1 -> Sum8/3

== system Orig_DSR_mod/CDOB_Subsys1/ND1/TimeDelayComp ==
  SysOut : Inport
  Dobsv : Inport  Port=2
  DelayCom : TransferFcn  Numerator=[a]  Denominator=[1 a 0]
  Sum8 : Sum  Inputs=|++
  FeedBack : Outport
  wires:
  DelayCom/1 -> Sum8/2
  SysOut/1 -> Sum8/1
  Sum8/1 -> FeedBack/1
  Dobsv/1 -> DelayCom/1

== system Orig_DSR_mod/CDOB_Subsys1/ND2/CDOB1 ==
  XRes : Inport
  Acc. : Inport  Port=2
  Derivative : Derivative  CoefficientInTFapproximation=0
  Gain : Gain  Gain=gnet/a
  Sum : Sum  Inputs=-+|
  Sum8 : Sum  Inputs=+-+
  Transfer Fcn2 : TransferFcn  Numerator=[gnet]  Denominator=[1 gnet]
  Dobsv : Outport
  wires:
  Transfer Fcn2/1 -> Sum/2
  Sum8/1 -> Transfer Fcn2/1
  Derivative/1 -> Sum8/2, Gain/1
  Gain/1 -> Sum8/1, Sum/1
  Sum/1 -> Dobsv/1
  XRes/1 -> Derivative/1
  Acc./1 -> Sum8/3

== system Orig_DSR_mod/CDOB_Subsys1/ND2/TimeDelayComp ==
  SysOut : Inport
  Dobsv : Inport  Port=2
  DelayCom : TransferFcn  Numerator=[a]  Denominator=[1 a 0]
  Sum8 : Sum  Inputs=|++
  FeedBack : Outport
  wires:
  DelayCom/1 -> Sum8/2
  SysOut/1 -> Sum8/1
  Sum8/1 -> FeedBack/1
  Dobsv/1 -> DelayCom/1

== system Orig_DSR_mod/CDOB_Subsys1/ND3/CDOB1 ==
  XRes : Inport
  Acc. : Inport  Port=2
  Derivative : Derivative  CoefficientInTFapproximation=0
  Gain : Gain  Gain=gnet/a
  Sum : Sum  Inputs=-+|
  Sum8 : Sum  Inputs=+-+
  Transfer Fcn2 : TransferFcn  Numerator=[gnet]  Denominator=[1 gnet]
  Dobsv : Outport
  wires:
  Transfer Fcn2/1 -> Sum/2
  Sum8/1 -> Transfer Fcn2/1
  Derivative/1 -> Sum8/2, Gain/1
  Gain/1 -> Sum8/1, Sum/1
  Sum/1 -> Dobsv/1
  XRes/1 -> Derivative/1
  Acc./1 -> Sum8/3

== system Orig_DSR_mod/CDOB_Subsys1/ND3/TimeDelayComp ==
  SysOut : Inport
  Dobsv : Inport  Port=2
  DelayCom : TransferFcn  Numerator=[a]  Denominator=[1 a 0]
  Sum8 : Sum  Inputs=|++
  FeedBack : Outport
  wires:
  DelayCom/1 -> Sum8/2
  SysOut/1 -> Sum8/1
  Sum8/1 -> FeedBack/1
  Dobsv/1 -> DelayCom/1

== system Orig_DSR_mod/CDOB_Subsys1/ND4/CDOB1 ==
  XRes : Inport
  Acc. : Inport  Port=2
  Derivative : Derivative  CoefficientInTFapproximation=0
  Gain : Gain  Gain=gnet/a
  Sum : Sum  Inputs=-+|
  Sum8 : Sum  Inputs=+-+
  Transfer Fcn2 : TransferFcn  Numerator=[gnet]  Denominator=[1 gnet]
  Dobsv : Outport
  wires:
  Transfer Fcn2/1 -> Sum/2
  Sum8/1 -> Transfer Fcn2/1
  Derivative/1 -> Sum8/2, Gain/1
  Gain/1 -> Sum8/1, Sum/1
  Sum/1 -> Dobsv/1
  XRes/1 -> Derivative/1
  Acc./1 -> Sum8/3

== system Orig_DSR_mod/CDOB_Subsys1/ND4/TimeDelayComp ==
  SysOut : Inport
  Dobsv : Inport  Port=2
  DelayCom : TransferFcn  Numerator=[a]  Denominator=[1 a 0]
  Sum8 : Sum  Inputs=|++
  FeedBack : Outport
  wires:
  DelayCom/1 -> Sum8/2
  SysOut/1 -> Sum8/1
  Sum8/1 -> FeedBack/1
  Dobsv/1 -> DelayCom/1

== system Orig_DSR_mod/CDOB_Subsys1/ND5/CDOB1 ==
  XRes : Inport
  Acc. : Inport  Port=2
  Derivative : Derivative  CoefficientInTFapproximation=0
  Gain : Gain  Gain=gnet/a
  Sum : Sum  Inputs=-+|
  Sum8 : Sum  Inputs=+-+
  Transfer Fcn2 : TransferFcn  Numerator=[gnet]  Denominator=[1 gnet]
  Dobsv : Outport
  wires:
  Transfer Fcn2/1 -> Sum/2
  Sum8/1 -> Transfer Fcn2/1
  Derivative/1 -> Sum8/2, Gain/1
  Gain/1 -> Sum8/1, Sum/1
  Sum/1 -> Dobsv/1
  XRes/1 -> Derivative/1
  Acc./1 -> Sum8/3

== system Orig_DSR_mod/CDOB_Subsys1/ND5/TimeDelayComp ==
  SysOut : Inport
  Dobsv : Inport  Port=2
  DelayCom : TransferFcn  Numerator=[a]  Denominator=[1 a 0]
  Sum8 : Sum  Inputs=|++
  FeedBack : Outport
  wires:
  DelayCom/1 -> Sum8/2
  SysOut/1 -> Sum8/1
  Sum8/1 -> FeedBack/1
  Dobsv/1 -> DelayCom/1

== system Orig_DSR_mod/CDOB_Subsys2/ND/CDOB1 ==
  XRes : Inport
  Acc. : Inport  Port=2
  Derivative : Derivative  CoefficientInTFapproximation=0
  Gain : Gain  Gain=gnet/a
  Sum : Sum  Inputs=-+|
  Sum8 : Sum  Inputs=+-+
  Transfer Fcn2 : TransferFcn  Numerator=[gnet]  Denominator=[1 gnet]
  Dobsv : Outport
  wires:
  Transfer Fcn2/1 -> Sum/2
  Sum8/1 -> Transfer Fcn2/1
  Derivative/1 -> Sum8/2, Gain/1
  Gain/1 -> Sum8/1, Sum/1
  Sum/1 -> Dobsv/1
  XRes/1 -> Derivative/1
  Acc./1 -> Sum8/3

== system Orig_DSR_mod/CDOB_Subsys2/ND/TimeDelayComp ==
  SysOut : Inport
  Dobsv : Inport  Port=2
  DelayCom : TransferFcn  Numerator=[a]  Denominator=[1 a 0]
  Sum8 : Sum  Inputs=|++
  FeedBack : Outport
  wires:
  DelayCom/1 -> Sum8/2
  SysOut/1 -> Sum8/1
  Sum8/1 -> FeedBack/1
  Dobsv/1 -> DelayCom/1

== system Orig_DSR_mod/CDOB_Subsys2/ND1/CDOB1 ==
  XRes : Inport
  Acc. : Inport  Port=2
  Derivative : Derivative  CoefficientInTFapproximation=0
  Gain : Gain  Gain=gnet/a
  Sum : Sum  Inputs=-+|
  Sum8 : Sum  Inputs=+-+
  Transfer Fcn2 : TransferFcn  Numerator=[gnet]  Denominator=[1 gnet]
  Dobsv : Outport
  wires:
  Transfer Fcn2/1 -> Sum/2
  Sum8/1 -> Transfer Fcn2/1
  Derivative/1 -> Sum8/2, Gain/1
  Gain/1 -> Sum8/1, Sum/1
  Sum/1 -> Dobsv/1
  XRes/1 -> Derivative/1
  Acc./1 -> Sum8/3

== system Orig_DSR_mod/CDOB_Subsys2/ND1/TimeDelayComp ==
  SysOut : Inport
  Dobsv : Inport  Port=2
  DelayCom : TransferFcn  Numerator=[a]  Denominator=[1 a 0]
  Sum8 : Sum  Inputs=|++
  FeedBack : Outport
  wires:
  DelayCom/1 -> Sum8/2
  SysOut/1 -> Sum8/1
  Sum8/1 -> FeedBack/1
  Dobsv/1 -> DelayCom/1

== system Orig_DSR_mod/CDOB_Subsys2/ND2/CDOB1 ==
  XRes : Inport
  Acc. : Inport  Port=2
  Derivative : Derivative  CoefficientInTFapproximation=0
  Gain : Gain  Gain=gnet/a
  Sum : Sum  Inputs=-+|
  Sum8 : Sum  Inputs=+-+
  Transfer Fcn2 : TransferFcn  Numerator=[gnet]  Denominator=[1 gnet]
  Dobsv : Outport
  wires:
  Transfer Fcn2/1 -> Sum/2
  Sum8/1 -> Transfer Fcn2/1
  Derivative/1 -> Sum8/2, Gain/1
  Gain/1 -> Sum8/1, Sum/1
  Sum/1 -> Dobsv/1
  XRes/1 -> Derivative/1
  Acc./1 -> Sum8/3

== system Orig_DSR_mod/CDOB_Subsys2/ND2/TimeDelayComp ==
  SysOut : Inport
  Dobsv : Inport  Port=2
  DelayCom : TransferFcn  Numerator=[a]  Denominator=[1 a 0]
  Sum8 : Sum  Inputs=|++
  FeedBack : Outport
  wires:
  DelayCom/1 -> Sum8/2
  SysOut/1 -> Sum8/1
  Sum8/1 -> FeedBack/1
  Dobsv/1 -> DelayCom/1

== system Orig_DSR_mod/CDOB_Subsys2/ND3/CDOB1 ==
  XRes : Inport
  Acc. : Inport  Port=2
  Derivative : Derivative  CoefficientInTFapproximation=0
  Gain : Gain  Gain=gnet/a
  Sum : Sum  Inputs=-+|
  Sum8 : Sum  Inputs=+-+
  Transfer Fcn2 : TransferFcn  Numerator=[gnet]  Denominator=[1 gnet]
  Dobsv : Outport
  wires:
  Transfer Fcn2/1 -> Sum/2
  Sum8/1 -> Transfer Fcn2/1
  Derivative/1 -> Sum8/2, Gain/1
  Gain/1 -> Sum8/1, Sum/1
  Sum/1 -> Dobsv/1
  XRes/1 -> Derivative/1
  Acc./1 -> Sum8/3

== system Orig_DSR_mod/CDOB_Subsys2/ND3/TimeDelayComp ==
  SysOut : Inport
  Dobsv : Inport  Port=2
  DelayCom : TransferFcn  Numerator=[a]  Denominator=[1 a 0]
  Sum8 : Sum  Inputs=|++
  FeedBack : Outport
  wires:
  DelayCom/1 -> Sum8/2
  SysOut/1 -> Sum8/1
  Sum8/1 -> FeedBack/1
  Dobsv/1 -> DelayCom/1

== system Orig_DSR_mod/CDOB_Subsys2/ND4/CDOB1 ==
  XRes : Inport
  Acc. : Inport  Port=2
  Derivative : Derivative  CoefficientInTFapproximation=0
  Gain : Gain  Gain=gnet/a
  Sum : Sum  Inputs=-+|
  Sum8 : Sum  Inputs=+-+
  Transfer Fcn2 : TransferFcn  Numerator=[gnet]  Denominator=[1 gnet]
  Dobsv : Outport
  wires:
  Transfer Fcn2/1 -> Sum/2
  Sum8/1 -> Transfer Fcn2/1
  Derivative/1 -> Sum8/2, Gain/1
  Gain/1 -> Sum8/1, Sum/1
  Sum/1 -> Dobsv/1
  XRes/1 -> Derivative/1
  Acc./1 -> Sum8/3

== system Orig_DSR_mod/CDOB_Subsys2/ND4/TimeDelayComp ==
  SysOut : Inport
  Dobsv : Inport  Port=2
  DelayCom : TransferFcn  Numerator=[a]  Denominator=[1 a 0]
  Sum8 : Sum  Inputs=|++
  FeedBack : Outport
  wires:
  DelayCom/1 -> Sum8/2
  SysOut/1 -> Sum8/1
  Sum8/1 -> FeedBack/1
  Dobsv/1 -> DelayCom/1

== system Orig_DSR_mod/CDOB_Subsys2/ND5/CDOB1 ==
  XRes : Inport
  Acc. : Inport  Port=2
  Derivative : Derivative  CoefficientInTFapproximation=0
  Gain : Gain  Gain=gnet/a
  Sum : Sum  Inputs=-+|
  Sum8 : Sum  Inputs=+-+
  Transfer Fcn2 : TransferFcn  Numerator=[gnet]  Denominator=[1 gnet]
  Dobsv : Outport
  wires:
  Transfer Fcn2/1 -> Sum/2
  Sum8/1 -> Transfer Fcn2/1
  Gain/1 -> Sum8/1, Sum/1
  Sum/1 -> Dobsv/1
  XRes/1 -> Derivative/1
  Acc./1 -> Sum8/3
  Derivative/1 -> Gain/1, Sum8/2

== system Orig_DSR_mod/CDOB_Subsys2/ND5/TimeDelayComp ==
  SysOut : Inport
  Dobsv : Inport  Port=2
  DelayCom : TransferFcn  Numerator=[a]  Denominator=[1 a 0]
  Sum8 : Sum  Inputs=|++
  FeedBack : Outport
  wires:
  DelayCom/1 -> Sum8/2
  SysOut/1 -> Sum8/1
  Sum8/1 -> FeedBack/1
  Dobsv/1 -> DelayCom/1

== system Orig_DSR_mod/CDOB_Subsys4/ND/CDOB1 ==
  XRes : Inport
  Acc. : Inport  Port=2
  Derivative : Derivative  CoefficientInTFapproximation=0
  Gain : Gain  Gain=gnet/a
  Sum : Sum  Inputs=-+|
  Sum8 : Sum  Inputs=+-+
  Transfer Fcn2 : TransferFcn  Numerator=[gnet]  Denominator=[1 gnet]
  Dobsv : Outport
  wires:
  Transfer Fcn2/1 -> Sum/2
  Sum8/1 -> Transfer Fcn2/1
  Derivative/1 -> Sum8/2, Gain/1
  Gain/1 -> Sum8/1, Sum/1
  Sum/1 -> Dobsv/1
  XRes/1 -> Derivative/1
  Acc./1 -> Sum8/3

== system Orig_DSR_mod/CDOB_Subsys4/ND/TimeDelayComp ==
  SysOut : Inport
  Dobsv : Inport  Port=2
  DelayCom : TransferFcn  Numerator=[a]  Denominator=[1 a 0]
  Sum8 : Sum  Inputs=|++
  FeedBack : Outport
  wires:
  DelayCom/1 -> Sum8/2
  SysOut/1 -> Sum8/1
  Sum8/1 -> FeedBack/1
  Dobsv/1 -> DelayCom/1

== system Orig_DSR_mod/CDOB_Subsys4/ND1/CDOB1 ==
  XRes : Inport
  Acc. : Inport  Port=2
  Derivative : Derivative  CoefficientInTFapproximation=0
  Gain : Gain  Gain=gnet/a
  Sum : Sum  Inputs=-+|
  Sum8 : Sum  Inputs=+-+
  Transfer Fcn2 : TransferFcn  Numerator=[gnet]  Denominator=[1 gnet]
  Dobsv : Outport
  wires:
  Transfer Fcn2/1 -> Sum/2
  Sum8/1 -> Transfer Fcn2/1
  Derivative/1 -> Sum8/2, Gain/1
  Gain/1 -> Sum8/1, Sum/1
  Sum/1 -> Dobsv/1
  XRes/1 -> Derivative/1
  Acc./1 -> Sum8/3

== system Orig_DSR_mod/CDOB_Subsys4/ND1/TimeDelayComp ==
  SysOut : Inport
  Dobsv : Inport  Port=2
  DelayCom : TransferFcn  Numerator=[a]  Denominator=[1 a 0]
  Sum8 : Sum  Inputs=|++
  FeedBack : Outport
  wires:
  DelayCom/1 -> Sum8/2
  SysOut/1 -> Sum8/1
  Sum8/1 -> FeedBack/1
  Dobsv/1 -> DelayCom/1

== system Orig_DSR_mod/CDOB_Subsys4/ND2/CDOB1 ==
  XRes : Inport
  Acc. : Inport  Port=2
  Derivative : Derivative  CoefficientInTFapproximation=0
  Gain : Gain  Gain=gnet/a
  Sum : Sum  Inputs=-+|
  Sum8 : Sum  Inputs=+-+
  Transfer Fcn2 : TransferFcn  Numerator=[gnet]  Denominator=[1 gnet]
  Dobsv : Outport
  wires:
  Transfer Fcn2/1 -> Sum/2
  Sum8/1 -> Transfer Fcn2/1
  Derivative/1 -> Sum8/2, Gain/1
  Gain/1 -> Sum8/1, Sum/1
  Sum/1 -> Dobsv/1
  XRes/1 -> Derivative/1
  Acc./1 -> Sum8/3

== system Orig_DSR_mod/CDOB_Subsys4/ND2/TimeDelayComp ==
  SysOut : Inport
  Dobsv : Inport  Port=2
  DelayCom : TransferFcn  Numerator=[a]  Denominator=[1 a 0]
  Sum8 : Sum  Inputs=|++
  FeedBack : Outport
  wires:
  DelayCom/1 -> Sum8/2
  SysOut/1 -> Sum8/1
  Sum8/1 -> FeedBack/1
  Dobsv/1 -> DelayCom/1

== system Orig_DSR_mod/CDOB_Subsys4/ND3/CDOB1 ==
  XRes : Inport
  Acc. : Inport  Port=2
  Derivative : Derivative  CoefficientInTFapproximation=0
  Gain : Gain  Gain=gnet/a
  Sum : Sum  Inputs=-+|
  Sum8 : Sum  Inputs=+-+
  Transfer Fcn2 : TransferFcn  Numerator=[gnet]  Denominator=[1 gnet]
  Dobsv : Outport
  wires:
  Transfer Fcn2/1 -> Sum/2
  Sum8/1 -> Transfer Fcn2/1
  Derivative/1 -> Sum8/2, Gain/1
  Gain/1 -> Sum8/1, Sum/1
  Sum/1 -> Dobsv/1
  XRes/1 -> Derivative/1
  Acc./1 -> Sum8/3

== system Orig_DSR_mod/CDOB_Subsys4/ND3/TimeDelayComp ==
  SysOut : Inport
  Dobsv : Inport  Port=2
  DelayCom : TransferFcn  Numerator=[a]  Denominator=[1 a 0]
  Sum8 : Sum  Inputs=|++
  FeedBack : Outport
  wires:
  DelayCom/1 -> Sum8/2
  SysOut/1 -> Sum8/1
  Sum8/1 -> FeedBack/1
  Dobsv/1 -> DelayCom/1

== system Orig_DSR_mod/CDOB_Subsys4/ND4/CDOB1 ==
  XRes : Inport
  Acc. : Inport  Port=2
  Derivative : Derivative  CoefficientInTFapproximation=0
  Gain : Gain  Gain=gnet/a
  Sum : Sum  Inputs=-+|
  Sum8 : Sum  Inputs=+-+
  Transfer Fcn2 : TransferFcn  Numerator=[gnet]  Denominator=[1 gnet]
  Dobsv : Outport
  wires:
  Transfer Fcn2/1 -> Sum/2
  Sum8/1 -> Transfer Fcn2/1
  Derivative/1 -> Sum8/2, Gain/1
  Gain/1 -> Sum8/1, Sum/1
  Sum/1 -> Dobsv/1
  XRes/1 -> Derivative/1
  Acc./1 -> Sum8/3

== system Orig_DSR_mod/CDOB_Subsys4/ND4/TimeDelayComp ==
  SysOut : Inport
  Dobsv : Inport  Port=2
  DelayCom : TransferFcn  Numerator=[a]  Denominator=[1 a 0]
  Sum8 : Sum  Inputs=|++
  FeedBack : Outport
  wires:
  DelayCom/1 -> Sum8/2
  SysOut/1 -> Sum8/1
  Sum8/1 -> FeedBack/1
  Dobsv/1 -> DelayCom/1

== system Orig_DSR_mod/CDOB_Subsys4/ND5/CDOB1 ==
  XRes : Inport
  Acc. : Inport  Port=2
  Derivative : Derivative  CoefficientInTFapproximation=0
  Gain : Gain  Gain=gnet/a
  Sum : Sum  Inputs=-+|
  Sum8 : Sum  Inputs=+-+
  Transfer Fcn2 : TransferFcn  Numerator=[gnet]  Denominator=[1 gnet]
  Dobsv : Outport
  wires:
  Transfer Fcn2/1 -> Sum/2
  Sum8/1 -> Transfer Fcn2/1
  Gain/1 -> Sum8/1, Sum/1
  Sum/1 -> Dobsv/1
  XRes/1 -> Derivative/1
  Acc./1 -> Sum8/3
  Derivative/1 -> Gain/1, Sum8/2

== system Orig_DSR_mod/CDOB_Subsys4/ND5/TimeDelayComp ==
  SysOut : Inport
  Dobsv : Inport  Port=2
  DelayCom : TransferFcn  Numerator=[a]  Denominator=[1 a 0]
  Sum8 : Sum  Inputs=|++
  FeedBack : Outport
  wires:
  DelayCom/1 -> Sum8/2
  SysOut/1 -> Sum8/1
  Sum8/1 -> FeedBack/1
  Dobsv/1 -> DelayCom/1

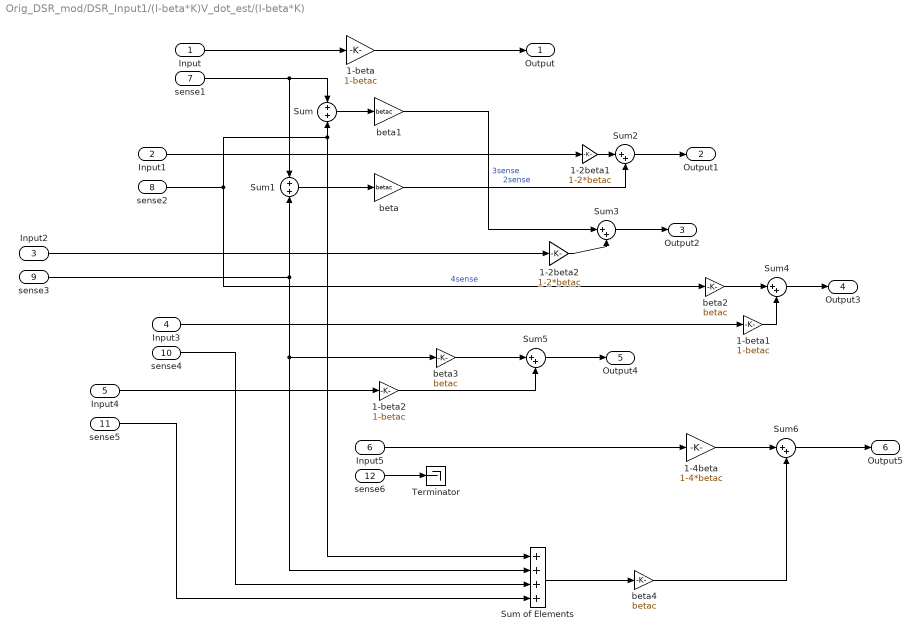
== system Orig_DSR_mod/DSR_Input1/(I-beta*K)V_dot_est/(I-beta*K) ==
  Input : Inport
  Input1 : Inport  Port=2
  Input2 : Inport  Port=3
  Input3 : Inport  Port=4
  Input4 : Inport  Port=5
  Input5 : Inport  Port=6
  sense1 : Inport  Port=7
  sense2 : Inport  Port=8
  sense3 : Inport  Port=9
  sense4 : Inport  Port=10
  sense5 : Inport  Port=11
  sense6 : Inport  Port=12
  1-2beta1 : Gain  Gain=1-2*betac
  1-2beta2 : Gain  Gain=1-2*betac
  1-4beta : Gain  Gain=1-4*betac
  1-beta : Gain  Gain=1-betac
  1-beta1 : Gain  Gain=1-betac
  1-beta2 : Gain  Gain=1-betac
  Sum : Sum  Inputs=+|+
  Sum of Elements : Sum  Inputs=++++
  Sum1 : Sum  Inputs=+|+
  Sum{2..6} (5 alike) : Sum  Inputs=|++
  Terminator : Terminator
  beta{,1..4} (5 alike) : Gain  Gain=betac
  Output : Outport
  Output1 : Outport  Port=2
  Output2 : Outport  Port=3
  Output3 : Outport  Port=4
  Output4 : Outport  Port=5
  Output5 : Outport  Port=6
  wires:
  Input/1 -> 1-beta/1
  1-2beta2/1 -> Sum3/2
  1-beta2/1 -> Sum5/2
  Sum4/1 -> Output3/1
  1-beta/1 -> Output/1
  beta/1 -> Sum2/2  "2sense"
  Sum6/1 -> Output5/1
  1-beta1/1 -> Sum4/2
  Input2/1 -> 1-2beta2/1
  1-2beta1/1 -> Sum2/1
  Input1/1 -> 1-2beta1/1
  beta4/1 -> Sum6/2
  Sum/1 -> beta1/1
  Input3/1 -> 1-beta1/1
  beta3/1 -> Sum5/1
  beta1/1 -> Sum3/1  "3sense"
  beta2/1 -> Sum4/1
  Sum5/1 -> Output4/1
  Input4/1 -> 1-beta2/1
  Sum1/1 -> beta/1
  1-4beta/1 -> Sum6/1
  Sum2/1 -> Output1/1
  Sum3/1 -> Output2/1
  Input5/1 -> 1-4beta/1
  Sum of Elements/1 -> beta4/1
  sense1/1 -> Sum1/1, Sum/1
  sense2/1 -> beta2/1, Sum of Elements/1, Sum/2  "4sense"
  sense3/1 -> beta3/1, Sum of Elements/2, Sum1/2
  sense5/1 -> Sum of Elements/4
  sense4/1 -> Sum of Elements/3
  sense6/1 -> Terminator/1

== system Orig_DSR_mod/DSR_Input1/(I-beta*K)V_dot_est/DerivativeEstimate ==
  pos : Inport
  pos1 : Inport  Port=2
  pos2 : Inport  Port=3
  pos3 : Inport  Port=4
  pos4 : Inport  Port=5
  pos5 : Inport  Port=6
  DSRdelayV1 : Subsystem
  DSRdelayV2 : Subsystem
  DSRdelayV3 : Subsystem
  DSRdelayV4 : Subsystem
  DSRdelayV5 : Subsystem
  DSRdelayV6 : Subsystem
  est : Outport
  est1 : Outport  Port=2
  est2 : Outport  Port=3
  est3 : Outport  Port=4
  est4 : Outport  Port=5
  est5 : Outport  Port=6
  wires:
  pos1/1 -> DSRdelayV1/1(Input)
  pos/1 -> DSRdelayV2/1(Input)
  DSRdelayV2/1(est) -> est/1
  pos2/1 -> DSRdelayV3/1(Input)
  pos3/1 -> DSRdelayV4/1(Input)
  pos4/1 -> DSRdelayV5/1(Input)
  pos5/1 -> DSRdelayV6/1(Input)
  DSRdelayV5/1(est) -> est4/1
  DSRdelayV6/1(est) -> est5/1
  DSRdelayV4/1(est) -> est3/1
  DSRdelayV3/1(est) -> est2/1
  DSRdelayV1/1(est) -> est1/1

== system Orig_DSR_mod/DSR_Input1/(I-beta*K)V_dot_est/DerivativeEstimate1 ==
  pos : Inport
  pos1 : Inport  Port=2
  pos2 : Inport  Port=3
  pos3 : Inport  Port=4
  pos4 : Inport  Port=5
  pos5 : Inport  Port=6
  DSRdelayV1 : Subsystem
  DSRdelayV2 : Subsystem
  DSRdelayV3 : Subsystem
  DSRdelayV4 : Subsystem
  DSRdelayV5 : Subsystem
  DSRdelayV6 : Subsystem
  est : Outport
  est1 : Outport  Port=2
  est2 : Outport  Port=3
  est3 : Outport  Port=4
  est4 : Outport  Port=5
  est5 : Outport  Port=6
  wires:
  pos1/1 -> DSRdelayV1/1(Input)
  pos/1 -> DSRdelayV2/1(Input)
  DSRdelayV2/1(est) -> est/1
  pos2/1 -> DSRdelayV3/1(Input)
  pos3/1 -> DSRdelayV4/1(Input)
  pos4/1 -> DSRdelayV5/1(Input)
  pos5/1 -> DSRdelayV6/1(Input)
  DSRdelayV5/1(est) -> est4/1
  DSRdelayV6/1(est) -> est5/1
  DSRdelayV4/1(est) -> est3/1
  DSRdelayV3/1(est) -> est2/1
  DSRdelayV1/1(est) -> est1/1

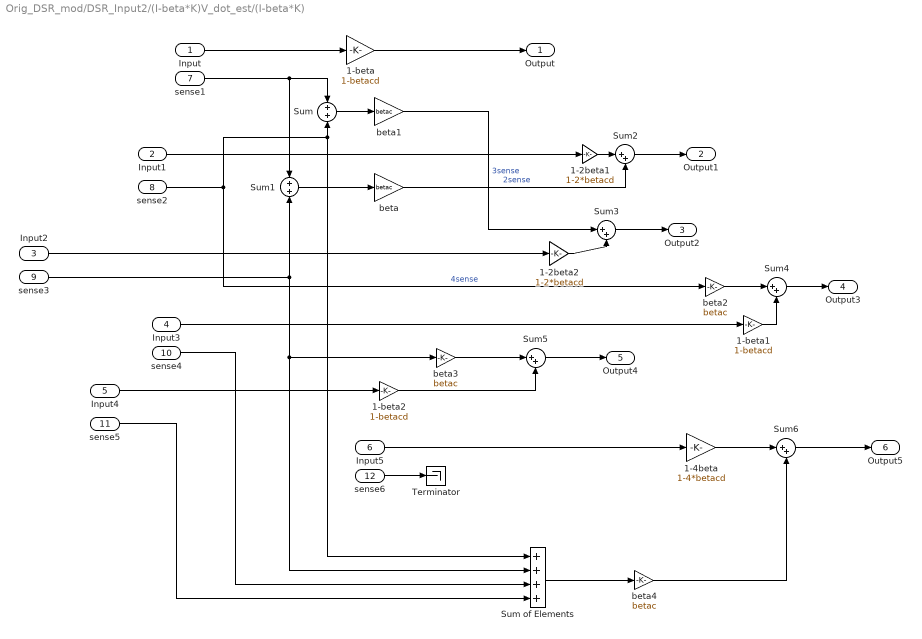
== system Orig_DSR_mod/DSR_Input2/(I-beta*K)V_dot_est/(I-beta*K) ==
  Input : Inport
  Input1 : Inport  Port=2
  Input2 : Inport  Port=3
  Input3 : Inport  Port=4
  Input4 : Inport  Port=5
  Input5 : Inport  Port=6
  sense1 : Inport  Port=7
  sense2 : Inport  Port=8
  sense3 : Inport  Port=9
  sense4 : Inport  Port=10
  sense5 : Inport  Port=11
  sense6 : Inport  Port=12
  1-2beta1 : Gain  Gain=1-2*betacd
  1-2beta2 : Gain  Gain=1-2*betacd
  1-4beta : Gain  Gain=1-4*betacd
  1-beta : Gain  Gain=1-betacd
  1-beta1 : Gain  Gain=1-betacd
  1-beta2 : Gain  Gain=1-betacd
  Sum : Sum  Inputs=+|+
  Sum of Elements : Sum  Inputs=++++
  Sum1 : Sum  Inputs=+|+
  Sum{2..6} (5 alike) : Sum  Inputs=|++
  Terminator : Terminator
  beta{,1..4} (5 alike) : Gain  Gain=betac
  Output : Outport
  Output1 : Outport  Port=2
  Output2 : Outport  Port=3
  Output3 : Outport  Port=4
  Output4 : Outport  Port=5
  Output5 : Outport  Port=6
  wires:
  Input/1 -> 1-beta/1
  1-2beta2/1 -> Sum3/2
  1-beta2/1 -> Sum5/2
  Sum4/1 -> Output3/1
  1-beta/1 -> Output/1
  beta/1 -> Sum2/2  "2sense"
  Sum6/1 -> Output5/1
  1-beta1/1 -> Sum4/2
  Input2/1 -> 1-2beta2/1
  1-2beta1/1 -> Sum2/1
  Input1/1 -> 1-2beta1/1
  beta4/1 -> Sum6/2
  Sum/1 -> beta1/1
  Input3/1 -> 1-beta1/1
  beta3/1 -> Sum5/1
  beta1/1 -> Sum3/1  "3sense"
  beta2/1 -> Sum4/1
  Sum5/1 -> Output4/1
  Input4/1 -> 1-beta2/1
  Sum1/1 -> beta/1
  1-4beta/1 -> Sum6/1
  Sum2/1 -> Output1/1
  Sum3/1 -> Output2/1
  Input5/1 -> 1-4beta/1
  Sum of Elements/1 -> beta4/1
  sense1/1 -> Sum1/1, Sum/1
  sense2/1 -> beta2/1, Sum of Elements/1, Sum/2  "4sense"
  sense3/1 -> beta3/1, Sum of Elements/2, Sum1/2
  sense5/1 -> Sum of Elements/4
  sense4/1 -> Sum of Elements/3
  sense6/1 -> Terminator/1

== system Orig_DSR_mod/DSR_Input2/(I-beta*K)V_dot_est/DerivativeEstimate ==
  pos : Inport
  pos1 : Inport  Port=2
  pos2 : Inport  Port=3
  pos3 : Inport  Port=4
  pos4 : Inport  Port=5
  pos5 : Inport  Port=6
  Derivative Estimator : Subsystem
  Derivative Estimator1 : Subsystem
  Derivative Estimator2 : Subsystem
  Derivative Estimator3 : Subsystem
  Derivative Estimator4 : Subsystem
  Derivative Estimator5 : Subsystem
  est : Outport
  est1 : Outport  Port=2
  est2 : Outport  Port=3
  est3 : Outport  Port=4
  est4 : Outport  Port=5
  est5 : Outport  Port=6
  wires:
  pos3/1 -> Derivative Estimator3/1(pos)
  Derivative Estimator4/1(est) -> est4/1
  Derivative Estimator2/1(est) -> est2/1
  Derivative Estimator3/1(est) -> est3/1
  Derivative Estimator1/1(est) -> est1/1
  pos1/1 -> Derivative Estimator1/1(pos)
  Derivative Estimator5/1(est) -> est5/1
  Derivative Estimator/1(est) -> est/1
  pos/1 -> Derivative Estimator/1(pos)
  pos2/1 -> Derivative Estimator2/1(pos)
  pos5/1 -> Derivative Estimator5/1(pos)
  pos4/1 -> Derivative Estimator4/1(pos)
